simulink model "Test7_withSimscapeBus"  (R2019b)
settings: Solver=VariableStepAuto  StartTime=0.0  StopTime=5  RelTol=1e-3
undefined symbols (not defined in the file): High, Low
libraries: fl_lib x49, nesl_utility x15, ee_lib x4, simulink x1
settings Model: Creator=lenovo  LastModifiedBy=czm6597
settings DebuggingCC: UnconnectedInputMsg=none  UnconnectedOutputMsg=none  UnconnectedLineMsg=none  SFMachineParentedDataDiag=error
settings ModelReferenceCC: EnableRefExpFcnMdlSchedulingChecks=off
settings RTWCC: Description=Generic Real-Time Target

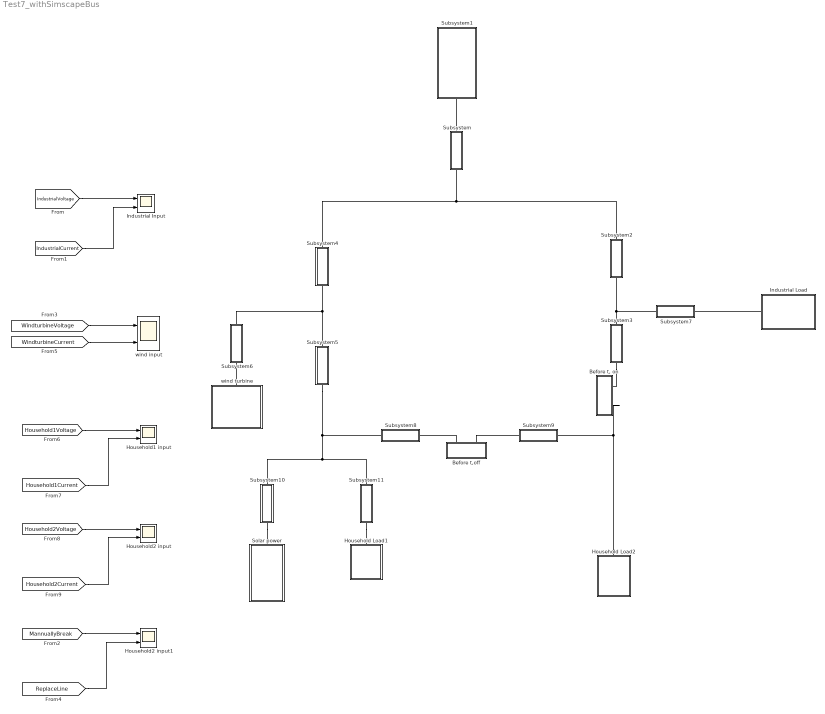
== system Test7_withSimscapeBus ==
  "Before t, on" : Subsystem  mask{t=3}
      mask prompts: t "Specific jumping time"
  Before t,off : Subsystem  mask{t=3}
      mask prompts: t "Specific jumping time"
  Household Load1 : Subsystem
  Household Load2 : Subsystem
  Household1 input : Scope  NumInputPorts=2
  Household2 input : Scope  NumInputPorts=2
  Household2 input1 : Scope  NumInputPorts=2
  Industrial Input : Scope  NumInputPorts=2
  Industrial Load : Subsystem
  Solar power : Subsystem
  Subsystem : Subsystem  mask{rho=1.68e-8, l=2.0, A=1.5e-6}
      mask prompts: rho "Specific resistivity in Ohm*m"; l "Length in m"; A "Cross sectional area in m^2"
  Subsystem1 : Subsystem
  Subsystem10 : Subsystem  mask{rho=1.68e-8, l=2.0, A=1.5e-6}
      mask prompts: rho "Specific resistivity in Ohm*m"; l "Length in m"; A "Cross sectional area in m^2"
  Subsystem11 : Subsystem  mask{rho=1.68e-8, l=2.0, A=1.5e-6}
      mask prompts: rho "Specific resistivity in Ohm*m"; l "Length in m"; A "Cross sectional area in m^2"
  Subsystem2 : Subsystem  mask{rho=1.68e-8, l=2.0, A=1.5e-6}
      mask prompts: rho "Specific resistivity in Ohm*m"; l "Length in m"; A "Cross sectional area in m^2"
  Subsystem3 : Subsystem  mask{rho=1.68e-8, l=2.0, A=1.5e-6}
      mask prompts: rho "Specific resistivity in Ohm*m"; l "Length in m"; A "Cross sectional area in m^2"
  Subsystem4 : Subsystem  mask{rho=1.68e-8, l=2.0, A=1.5e-6}
      mask prompts: rho "Specific resistivity in Ohm*m"; l "Length in m"; A "Cross sectional area in m^2"
  Subsystem5 : Subsystem  mask{rho=1.68e-8, l=2.0, A=1.5e-6}
      mask prompts: rho "Specific resistivity in Ohm*m"; l "Length in m"; A "Cross sectional area in m^2"
  Subsystem6 : Subsystem  mask{rho=1.68e-8, l=2.0, A=1.5e-6}
      mask prompts: rho "Specific resistivity in Ohm*m"; l "Length in m"; A "Cross sectional area in m^2"
  Subsystem7 : Subsystem  mask{rho=1.68e-8, l=2.0, A=1.5e-6}
      mask prompts: rho "Specific resistivity in Ohm*m"; l "Length in m"; A "Cross sectional area in m^2"
  Subsystem8 : Subsystem  mask{rho=1.68e-8, l=2.0, A=1.5e-6}
      mask prompts: rho "Specific resistivity in Ohm*m"; l "Length in m"; A "Cross sectional area in m^2"
  Subsystem9 : Subsystem  mask{rho=1.68e-8, l=2.0, A=1.5e-6}
      mask prompts: rho "Specific resistivity in Ohm*m"; l "Length in m"; A "Cross sectional area in m^2"
  wind input : Scope  NumInputPorts=2
  wind turbine : Subsystem
  wires:
  [Household2Current] -> Household2 input/2
  [Household2Voltage] -> Household2 input/1
  [Household1Current] -> Household1 input/2
  [Household1Voltage] -> Household1 input/1
  [WindturbineCurrent] -> wind input/2
  [IndustrialCurrent] -> Industrial Input/2
  [IndustrialVoltage] -> Industrial Input/1
  [WindturbineVoltage] -> wind input/1
  [MannuallyBreak] -> Household2 input1/1
  [ReplaceLine] -> Household2 input1/2
  connections:
  Subsystem/RConn1 -- Subsystem4/LConn1 -- Subsystem2/LConn1
  Subsystem/LConn1 -- Subsystem1/RConn1
  Subsystem3/LConn1 -- Subsystem7/LConn1 -- Subsystem2/RConn1
  Subsystem5/LConn1 -- Subsystem6/RConn1 -- Subsystem4/RConn1
  wind turbine/LConn1 -- Subsystem6/LConn1
  Industrial Load/RConn1 -- Subsystem7/RConn1
  Subsystem5/RConn1 -- Subsystem11/LConn1 -- Subsystem10/LConn1 -- Subsystem8/RConn1
  Subsystem11/RConn1 -- Household Load1/LConn1
  Subsystem10/RConn1 -- Solar power/LConn1
  Subsystem3/RConn1 -- "Before t, on"/LConn1
  "Before t, on"/LConn2 -- Household Load2/LConn1 -- Subsystem9/LConn1
  Before t,off/LConn1 -- Subsystem8/LConn1
  Before t,off/LConn2 -- Subsystem9/RConn1

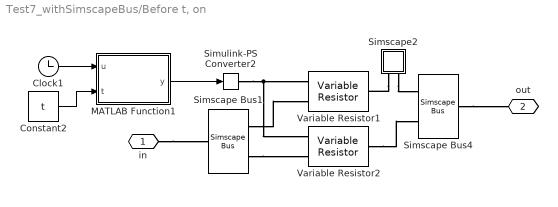
== system Test7_withSimscapeBus/Before t, on ==
  Clock1 : Clock
  Constant2 : Constant  Value=t
  MATLAB Function1 : MATLAB Function  TreatAsAtomicUnit=on
  Simscape Bus1 : SimscapeBus  HierarchyStrings=High;Low
  Simscape Bus4 : SimscapeBus  HierarchyStrings=High;Low
  Simscape2 : Subsystem
      mask Display:
      | disp('A')
      | port_label('LConn',1,'+')
      | port_label('LConn',2,'-')
  Simulink-PS Converter2 : nesl_utility/Simulink-PS Converter  PhysicalDomain=network_engine_domain  SubClassName=ps_input  LeftPortType=input  RightPortType=output  PseudoPeriodic=off  Frequencies=[]  NoiseDistribution=none  NoiseParameters=[]  Unit=1  AffineConversion=off  FilteringAndDerivatives=provide  SimscapeFilterOrder=1  InputFilterTimeConstant=0.001  UdotUserProvided=0
  Variable Resistor1 : fl_lib/Electrical/Electrical Elements/Variable Resistor  Rmin=0 Ohm  i_specify=off  i_priority=None  i=0 A  i_nominal_specify=off  i_nominal_unit=A  i_nominal_value=1  v_specify=off  v_priority=None  v=0 V  v_nominal_specify=off  v_nominal_unit=V  v_nominal_value=1
  Variable Resistor2 : fl_lib/Electrical/Electrical Elements/Variable Resistor  Rmin=0 Ohm  i_specify=off  i_priority=None  i=0 A  i_nominal_specify=off  i_nominal_unit=A  i_nominal_value=1  v_specify=off  v_priority=None  v=0 V  v_nominal_specify=off  v_nominal_unit=V  v_nominal_value=1
  in : PMIOPort  Side=Left
  out : PMIOPort  Port=2  Side=Left
  wires:
  Clock1/1 -> MATLAB Function1/1(u)
  Constant2/1 -> MATLAB Function1/2(t)
  MATLAB Function1/1(y) -> Simulink-PS Converter2/1
  connections:
  Simscape2/LConn1 -- Variable Resistor1/RConn1
  Simulink-PS Converter2/RConn1 -- Variable Resistor1/LConn1 -- Variable Resistor2/LConn1
  in/RConn1 -- Simscape Bus1/RConn1
  Simscape Bus1/LConn2 -- Variable Resistor2/LConn2
  Simscape Bus1/LConn1 -- Variable Resistor1/LConn2
  Variable Resistor2/RConn1 -- Simscape Bus4/LConn2
  Simscape Bus4/RConn1 -- out/RConn1
  Simscape2/LConn2 -- Simscape Bus4/LConn1

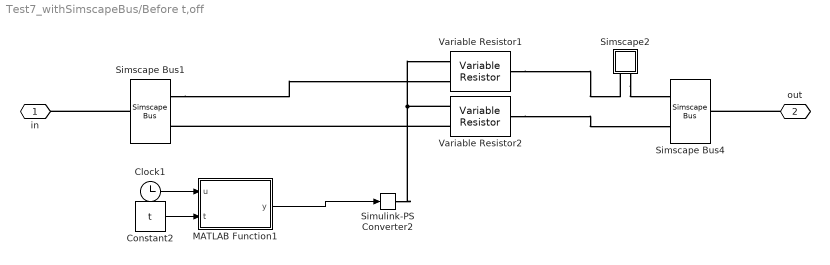
== system Test7_withSimscapeBus/Before t,off ==
  Clock1 : Clock
  Constant2 : Constant  Value=t
  MATLAB Function1 : MATLAB Function  TreatAsAtomicUnit=on
  Simscape Bus1 : SimscapeBus  HierarchyStrings=High;Low
  Simscape Bus4 : SimscapeBus  HierarchyStrings=High;Low
  Simscape2 : Subsystem
      mask Display:
      | disp('A')
      | port_label('LConn',1,'+')
      | port_label('LConn',2,'-')
  Simulink-PS Converter2 : nesl_utility/Simulink-PS Converter  PhysicalDomain=network_engine_domain  SubClassName=ps_input  LeftPortType=input  RightPortType=output  PseudoPeriodic=off  Frequencies=[]  NoiseDistribution=none  NoiseParameters=[]  Unit=1  AffineConversion=off  FilteringAndDerivatives=provide  SimscapeFilterOrder=1  InputFilterTimeConstant=0.001  UdotUserProvided=0
  Variable Resistor1 : fl_lib/Electrical/Electrical Elements/Variable Resistor  Rmin=0 Ohm  i_specify=off  i_priority=None  i=0 A  i_nominal_specify=off  i_nominal_unit=A  i_nominal_value=1  v_specify=off  v_priority=None  v=0 V  v_nominal_specify=off  v_nominal_unit=V  v_nominal_value=1
  Variable Resistor2 : fl_lib/Electrical/Electrical Elements/Variable Resistor  Rmin=0 Ohm  i_specify=off  i_priority=None  i=0 A  i_nominal_specify=off  i_nominal_unit=A  i_nominal_value=1  v_specify=off  v_priority=None  v=0 V  v_nominal_specify=off  v_nominal_unit=V  v_nominal_value=1
  in : PMIOPort  Side=Left
  out : PMIOPort  Port=2  Side=Left
  wires:
  MATLAB Function1/1(y) -> Simulink-PS Converter2/1
  Constant2/1 -> MATLAB Function1/2(t)
  Clock1/1 -> MATLAB Function1/1(u)
  connections:
  out/RConn1 -- Simscape Bus4/RConn1
  Simscape Bus1/RConn1 -- in/RConn1
  Variable Resistor2/LConn2 -- Simscape Bus1/LConn2
  Simscape Bus1/LConn1 -- Variable Resistor1/LConn2
  Variable Resistor1/RConn1 -- Simscape2/LConn1
  Variable Resistor2/RConn1 -- Simscape Bus4/LConn2
  Simulink-PS Converter2/RConn1 -- Variable Resistor1/LConn1 -- Variable Resistor2/LConn1
  Simscape2/LConn2 -- Simscape Bus4/LConn1

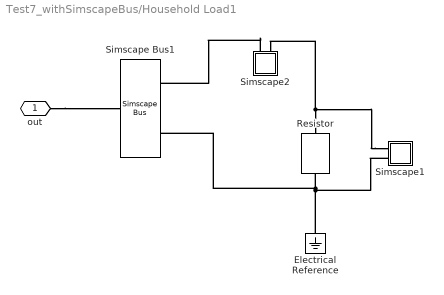
== system Test7_withSimscapeBus/Household Load1 ==
  Electrical Reference : fl_lib/Electrical/Electrical Elements/Electrical Reference
  Resistor : fl_lib/Electrical/Electrical Elements/Resistor  R=1 Ohm  i_specify=off  i_priority=None  i=0 A  i_nominal_specify=off  i_nominal_unit=A  i_nominal_value=1  v_specify=off  v_priority=None  v=0 V  v_nominal_specify=off  v_nominal_unit=V  v_nominal_value=1
  Simscape Bus1 : SimscapeBus  HierarchyStrings=High;Low
  Simscape1 : Subsystem
      mask Display:
      | disp('V')
      | port_label('LConn',1,'+')
      | port_label('LConn',2,'-')
  Simscape2 : Subsystem
      mask Display:
      | disp('A')
      | port_label('LConn',1,'+')
      | port_label('LConn',2,'-')
  out : PMIOPort  Side=Left
  connections:
  Simscape2/LConn1 -- Simscape Bus1/LConn1
  Simscape1/LConn1 -- Simscape2/LConn2 -- Resistor/LConn1
  Simscape1/LConn2 -- Simscape Bus1/LConn2 -- Resistor/RConn1 -- Electrical Reference/LConn1
  out/RConn1 -- Simscape Bus1/RConn1

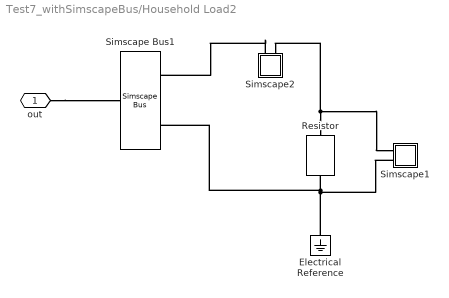
== system Test7_withSimscapeBus/Household Load2 ==
  Electrical Reference : fl_lib/Electrical/Electrical Elements/Electrical Reference
  Resistor : fl_lib/Electrical/Electrical Elements/Resistor  R=1 Ohm  i_specify=off  i_priority=None  i=0 A  i_nominal_specify=off  i_nominal_unit=A  i_nominal_value=1  v_specify=off  v_priority=None  v=0 V  v_nominal_specify=off  v_nominal_unit=V  v_nominal_value=1
  Simscape Bus1 : SimscapeBus  HierarchyStrings=High;Low
  Simscape1 : Subsystem
      mask Display:
      | disp('V')
      | port_label('LConn',1,'+')
      | port_label('LConn',2,'-')
  Simscape2 : Subsystem
      mask Display:
      | disp('A')
      | port_label('LConn',1,'+')
      | port_label('LConn',2,'-')
  out : PMIOPort  Side=Left
  connections:
  Electrical Reference/LConn1 -- Simscape Bus1/LConn2 -- Resistor/RConn1 -- Simscape1/LConn2
  Resistor/LConn1 -- Simscape2/LConn2 -- Simscape1/LConn1
  Simscape2/LConn1 -- Simscape Bus1/LConn1
  out/RConn1 -- Simscape Bus1/RConn1

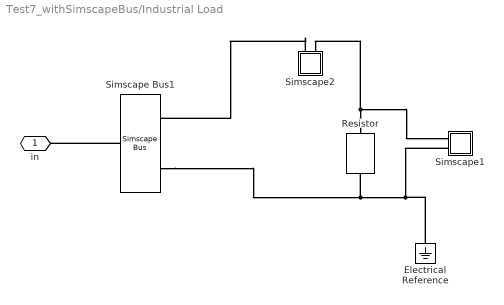
== system Test7_withSimscapeBus/Industrial Load ==
  Electrical Reference : fl_lib/Electrical/Electrical Elements/Electrical Reference
  Resistor : fl_lib/Electrical/Electrical Elements/Resistor  R=1 Ohm  i_specify=off  i_priority=None  i=0 A  i_nominal_specify=off  i_nominal_unit=A  i_nominal_value=1  v_specify=off  v_priority=None  v=0 V  v_nominal_specify=off  v_nominal_unit=V  v_nominal_value=1
  Simscape Bus1 : SimscapeBus  HierarchyStrings=High;Low
  Simscape1 : Subsystem
      mask Display:
      | disp('V')
      | port_label('LConn',1,'+')
      | port_label('LConn',2,'-')
  Simscape2 : Subsystem
      mask Display:
      | disp('A')
      | port_label('LConn',1,'+')
      | port_label('LConn',2,'-')
  in : PMIOPort  Side=Right
  connections:
  Simscape2/LConn1 -- Simscape Bus1/LConn1
  Simscape Bus1/RConn1 -- in/RConn1
  Resistor/LConn1 -- Simscape2/LConn2 -- Simscape1/LConn1
  Electrical Reference/LConn1 -- Simscape Bus1/LConn2 -- Resistor/RConn1 -- Simscape1/LConn2

== system Test7_withSimscapeBus/Solar power ==
  Current Source1 : ee_lib/Sources/Current Source  dc_current=0.6 A  ac_current=0 A  ac_shift=0 rad  ac_frequency=60 Hz  noise_mode=0  PSD=0 A^2/Hz  repeatability=1  auto_seed=2280044724  user_seed=0  sample_time=1e-3 s  i_specify=off  i_priority=None  i=0 A  i_nominal_specify=off  i_nominal_unit=A  i_nominal_value=1  v_specify=off  v_priority=None  v=0 V  v_nominal_specify=off  v_nominal_unit=V  v_nominal_value=1
      settings: SourceProductName=Simscape Electrical  SourceProductBaseCode=PS
  Resistor : ee_lib/Passive/Resistor  R=0.3 Ohm  R_tol=5  enable_R_tol=0  tol_distribution=1  nSigma=4  enable_operating_limits=0  operating_limit_action=2  max_working_voltage=100 V  power_rating=1 W  enable_faults=0  fault_action=1  R_faulted=inf Ohm  enable_temporal_fault=0  t_fault=1 s  enable_behavioral_fault=0  max_permissible_current=1 A  t_fail_on_current=1 s  noise_mode=0  sample_time=1e-3 s  repeatability=1  auto_seed=2715962282  user_seed=0  Tdevice=25 degC  alpha=3.93e-3 1/K  Tmeas=25 degC  thermal_mass=100 J/K  power_derating_T1=70 degC  power_derating_T2=155 degC  operating_temperature_range_vec=[-50, 150] degC  temperature_specify=off  temperature_priority=High  temperature=298.15 K  temperature_nominal_specify=off  temperature_nominal_unit=K  temperature_nominal_value=1
      settings: SourceProductName=Simscape Electrical
  Simscape Bus1 : SimscapeBus  HierarchyStrings=High;Low
  out : PMIOPort  Side=Left
  connections:
  Simscape Bus1/LConn1 -- Current Source1/LConn1 -- Resistor/LConn1
  Resistor/RConn1 -- Current Source1/RConn1 -- Simscape Bus1/LConn2
  out/RConn1 -- Simscape Bus1/RConn1

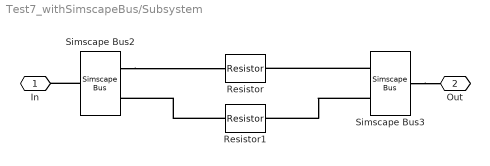
== system Test7_withSimscapeBus/Subsystem ==
  Resistor : fl_lib/Electrical/Electrical Elements/Resistor  R=rho*l/A Ohm  i_specify=off  i_priority=None  i=0 A  i_nominal_specify=off  i_nominal_unit=A  i_nominal_value=1  v_specify=off  v_priority=None  v=0 V  v_nominal_specify=off  v_nominal_unit=V  v_nominal_value=1
  Resistor1 : fl_lib/Electrical/Electrical Elements/Resistor  R=rho*l/A Ohm  i_specify=off  i_priority=None  i=0 A  i_nominal_specify=off  i_nominal_unit=A  i_nominal_value=1  v_specify=off  v_priority=None  v=0 V  v_nominal_specify=off  v_nominal_unit=V  v_nominal_value=1
  Simscape Bus2 : SimscapeBus  HierarchyStrings=High;Low
  Simscape Bus3 : SimscapeBus  HierarchyStrings=High;Low
  In : PMIOPort  Side=Left
  Out : PMIOPort  Port=2  Side=Right
  connections:
  Simscape Bus2/LConn1 -- Resistor/LConn1
  Simscape Bus3/LConn2 -- Resistor1/RConn1
  Simscape Bus2/RConn1 -- In/RConn1
  Simscape Bus3/LConn1 -- Resistor/RConn1
  Resistor1/LConn1 -- Simscape Bus2/LConn2
  Simscape Bus3/RConn1 -- Out/RConn1

== system Test7_withSimscapeBus/Subsystem1 ==
  note: DC voltage source
  note: DLP: DC line parameter
  DC Voltage Source1 : ee_lib/Additional Components/SPICE Sources/DC Voltage Source  DC=5 V
      settings: SourceProductName=Simscape Electrical
  Electrical Reference1 : fl_lib/Electrical/Electrical Elements/Electrical Reference
  Simscape Bus : SimscapeBus  HierarchyStrings=High;Low
  Solver Configuration1 : nesl_utility/Solver Configuration  PhysicalDomain=network_engine_domain  SubClassName=solver  LeftPortType=input  RightPortType=generic  Tones=[]  Harmonics=[]  SimulateNoise=off  Profile=off  UseLocalSampling=off  EnableSwitchedLinearOptims=on  FrequencyDomain=off  UseCCode=off  RelTol=0.001  AbsTol=1e-06  MinStep=1e-09  ToWorkspace=off  RevertToSquareIcSolve=off  NumHomotopyIterations=100  PhasorMode=off  PhasorModeNumHarmonics=1  DoDC=off  ResidualTolerance=1e-9  UseLocalSolver=on  LocalSolverChoice=NE_BACKWARD_EULER_ADVANCER  LocalSolverSampleTime=5e-6  DoFixedCost=on  MaxNonlinIter=3  MaxModeIter=2  LinearAlgebra=auto  EquationFormulation=NE_TIME_EF  DelaysMemoryBudget=1024  AutomaticFiltering=on  FilteringTimeConstant=0.001  PartitionStorageMethod=AS_NEEDED  PartitionMemoryBudget=1024  PartitionMethod=FAST
  out : PMIOPort  Side=Right
  connections:
  DC Voltage Source1/LConn1 -- Simscape Bus/LConn1
  DC Voltage Source1/RConn1 -- Simscape Bus/LConn2 -- Electrical Reference1/LConn1 -- Solver Configuration1/RConn1
  out/RConn1 -- Simscape Bus/RConn1

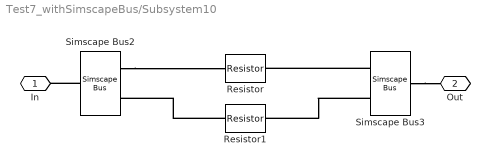
== system Test7_withSimscapeBus/Subsystem10 ==
  Resistor : fl_lib/Electrical/Electrical Elements/Resistor  R=rho*l/A Ohm  i_specify=off  i_priority=None  i=0 A  i_nominal_specify=off  i_nominal_unit=A  i_nominal_value=1  v_specify=off  v_priority=None  v=0 V  v_nominal_specify=off  v_nominal_unit=V  v_nominal_value=1
  Resistor1 : fl_lib/Electrical/Electrical Elements/Resistor  R=rho*l/A Ohm  i_specify=off  i_priority=None  i=0 A  i_nominal_specify=off  i_nominal_unit=A  i_nominal_value=1  v_specify=off  v_priority=None  v=0 V  v_nominal_specify=off  v_nominal_unit=V  v_nominal_value=1
  Simscape Bus2 : SimscapeBus  HierarchyStrings=High;Low
  Simscape Bus3 : SimscapeBus  HierarchyStrings=High;Low
  In : PMIOPort  Side=Left
  Out : PMIOPort  Port=2  Side=Right
  connections:
  Simscape Bus3/RConn1 -- Out/RConn1
  Resistor1/LConn1 -- Simscape Bus2/LConn2
  Simscape Bus3/LConn1 -- Resistor/RConn1
  Simscape Bus2/RConn1 -- In/RConn1
  Simscape Bus3/LConn2 -- Resistor1/RConn1
  Simscape Bus2/LConn1 -- Resistor/LConn1

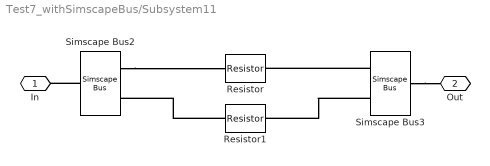
== system Test7_withSimscapeBus/Subsystem11 ==
  Resistor : fl_lib/Electrical/Electrical Elements/Resistor  R=rho*l/A Ohm  i_specify=off  i_priority=None  i=0 A  i_nominal_specify=off  i_nominal_unit=A  i_nominal_value=1  v_specify=off  v_priority=None  v=0 V  v_nominal_specify=off  v_nominal_unit=V  v_nominal_value=1
  Resistor1 : fl_lib/Electrical/Electrical Elements/Resistor  R=rho*l/A Ohm  i_specify=off  i_priority=None  i=0 A  i_nominal_specify=off  i_nominal_unit=A  i_nominal_value=1  v_specify=off  v_priority=None  v=0 V  v_nominal_specify=off  v_nominal_unit=V  v_nominal_value=1
  Simscape Bus2 : SimscapeBus  HierarchyStrings=High;Low
  Simscape Bus3 : SimscapeBus  HierarchyStrings=High;Low
  In : PMIOPort  Side=Left
  Out : PMIOPort  Port=2  Side=Right
  connections:
  Simscape Bus2/LConn1 -- Resistor/LConn1
  Simscape Bus3/LConn2 -- Resistor1/RConn1
  Simscape Bus2/RConn1 -- In/RConn1
  Simscape Bus3/LConn1 -- Resistor/RConn1
  Resistor1/LConn1 -- Simscape Bus2/LConn2
  Simscape Bus3/RConn1 -- Out/RConn1

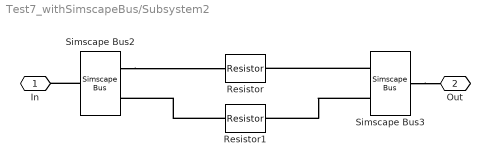
== system Test7_withSimscapeBus/Subsystem2 ==
  Resistor : fl_lib/Electrical/Electrical Elements/Resistor  R=rho*l/A Ohm  i_specify=off  i_priority=None  i=0 A  i_nominal_specify=off  i_nominal_unit=A  i_nominal_value=1  v_specify=off  v_priority=None  v=0 V  v_nominal_specify=off  v_nominal_unit=V  v_nominal_value=1
  Resistor1 : fl_lib/Electrical/Electrical Elements/Resistor  R=rho*l/A Ohm  i_specify=off  i_priority=None  i=0 A  i_nominal_specify=off  i_nominal_unit=A  i_nominal_value=1  v_specify=off  v_priority=None  v=0 V  v_nominal_specify=off  v_nominal_unit=V  v_nominal_value=1
  Simscape Bus2 : SimscapeBus  HierarchyStrings=High;Low
  Simscape Bus3 : SimscapeBus  HierarchyStrings=High;Low
  In : PMIOPort  Side=Left
  Out : PMIOPort  Port=2  Side=Right
  connections:
  Simscape Bus3/RConn1 -- Out/RConn1
  Resistor1/LConn1 -- Simscape Bus2/LConn2
  Simscape Bus3/LConn1 -- Resistor/RConn1
  Simscape Bus2/RConn1 -- In/RConn1
  Simscape Bus3/LConn2 -- Resistor1/RConn1
  Simscape Bus2/LConn1 -- Resistor/LConn1

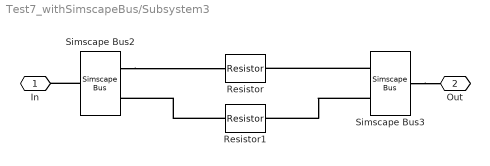
== system Test7_withSimscapeBus/Subsystem3 ==
  Resistor : fl_lib/Electrical/Electrical Elements/Resistor  R=rho*l/A Ohm  i_specify=off  i_priority=None  i=0 A  i_nominal_specify=off  i_nominal_unit=A  i_nominal_value=1  v_specify=off  v_priority=None  v=0 V  v_nominal_specify=off  v_nominal_unit=V  v_nominal_value=1
  Resistor1 : fl_lib/Electrical/Electrical Elements/Resistor  R=rho*l/A Ohm  i_specify=off  i_priority=None  i=0 A  i_nominal_specify=off  i_nominal_unit=A  i_nominal_value=1  v_specify=off  v_priority=None  v=0 V  v_nominal_specify=off  v_nominal_unit=V  v_nominal_value=1
  Simscape Bus2 : SimscapeBus  HierarchyStrings=High;Low
  Simscape Bus3 : SimscapeBus  HierarchyStrings=High;Low
  In : PMIOPort  Side=Left
  Out : PMIOPort  Port=2  Side=Right
  connections:
  Simscape Bus3/RConn1 -- Out/RConn1
  Resistor1/LConn1 -- Simscape Bus2/LConn2
  Simscape Bus3/LConn1 -- Resistor/RConn1
  Simscape Bus2/RConn1 -- In/RConn1
  Simscape Bus3/LConn2 -- Resistor1/RConn1
  Simscape Bus2/LConn1 -- Resistor/LConn1

== system Test7_withSimscapeBus/Subsystem4 ==
  Resistor : fl_lib/Electrical/Electrical Elements/Resistor  R=rho*l/A Ohm  i_specify=off  i_priority=None  i=0 A  i_nominal_specify=off  i_nominal_unit=A  i_nominal_value=1  v_specify=off  v_priority=None  v=0 V  v_nominal_specify=off  v_nominal_unit=V  v_nominal_value=1
  Resistor1 : fl_lib/Electrical/Electrical Elements/Resistor  R=rho*l/A Ohm  i_specify=off  i_priority=None  i=0 A  i_nominal_specify=off  i_nominal_unit=A  i_nominal_value=1  v_specify=off  v_priority=None  v=0 V  v_nominal_specify=off  v_nominal_unit=V  v_nominal_value=1
  Simscape Bus2 : SimscapeBus  HierarchyStrings=High;Low
  Simscape Bus3 : SimscapeBus  HierarchyStrings=High;Low
  In : PMIOPort  Side=Left
  Out : PMIOPort  Port=2  Side=Right
  connections:
  Simscape Bus3/RConn1 -- Out/RConn1
  Resistor1/LConn1 -- Simscape Bus2/LConn2
  Simscape Bus3/LConn1 -- Resistor/RConn1
  Simscape Bus2/RConn1 -- In/RConn1
  Simscape Bus3/LConn2 -- Resistor1/RConn1
  Simscape Bus2/LConn1 -- Resistor/LConn1

== system Test7_withSimscapeBus/Subsystem5 ==
  Resistor : fl_lib/Electrical/Electrical Elements/Resistor  R=rho*l/A Ohm  i_specify=off  i_priority=None  i=0 A  i_nominal_specify=off  i_nominal_unit=A  i_nominal_value=1  v_specify=off  v_priority=None  v=0 V  v_nominal_specify=off  v_nominal_unit=V  v_nominal_value=1
  Resistor1 : fl_lib/Electrical/Electrical Elements/Resistor  R=rho*l/A Ohm  i_specify=off  i_priority=None  i=0 A  i_nominal_specify=off  i_nominal_unit=A  i_nominal_value=1  v_specify=off  v_priority=None  v=0 V  v_nominal_specify=off  v_nominal_unit=V  v_nominal_value=1
  Simscape Bus2 : SimscapeBus  HierarchyStrings=High;Low
  Simscape Bus3 : SimscapeBus  HierarchyStrings=High;Low
  In : PMIOPort  Side=Left
  Out : PMIOPort  Port=2  Side=Right
  connections:
  Simscape Bus2/LConn1 -- Resistor/LConn1
  Simscape Bus3/LConn2 -- Resistor1/RConn1
  Simscape Bus2/RConn1 -- In/RConn1
  Simscape Bus3/LConn1 -- Resistor/RConn1
  Resistor1/LConn1 -- Simscape Bus2/LConn2
  Simscape Bus3/RConn1 -- Out/RConn1

== system Test7_withSimscapeBus/Subsystem6 ==
  Resistor : fl_lib/Electrical/Electrical Elements/Resistor  R=rho*l/A Ohm  i_specify=off  i_priority=None  i=0 A  i_nominal_specify=off  i_nominal_unit=A  i_nominal_value=1  v_specify=off  v_priority=None  v=0 V  v_nominal_specify=off  v_nominal_unit=V  v_nominal_value=1
  Resistor1 : fl_lib/Electrical/Electrical Elements/Resistor  R=rho*l/A Ohm  i_specify=off  i_priority=None  i=0 A  i_nominal_specify=off  i_nominal_unit=A  i_nominal_value=1  v_specify=off  v_priority=None  v=0 V  v_nominal_specify=off  v_nominal_unit=V  v_nominal_value=1
  Simscape Bus2 : SimscapeBus  HierarchyStrings=High;Low
  Simscape Bus3 : SimscapeBus  HierarchyStrings=High;Low
  In : PMIOPort  Side=Left
  Out : PMIOPort  Port=2  Side=Right
  connections:
  Simscape Bus2/LConn1 -- Resistor/LConn1
  Simscape Bus3/LConn2 -- Resistor1/RConn1
  Simscape Bus2/RConn1 -- In/RConn1
  Simscape Bus3/LConn1 -- Resistor/RConn1
  Resistor1/LConn1 -- Simscape Bus2/LConn2
  Simscape Bus3/RConn1 -- Out/RConn1

== system Test7_withSimscapeBus/Subsystem7 ==
  Resistor : fl_lib/Electrical/Electrical Elements/Resistor  R=rho*l/A Ohm  i_specify=off  i_priority=None  i=0 A  i_nominal_specify=off  i_nominal_unit=A  i_nominal_value=1  v_specify=off  v_priority=None  v=0 V  v_nominal_specify=off  v_nominal_unit=V  v_nominal_value=1
  Resistor1 : fl_lib/Electrical/Electrical Elements/Resistor  R=rho*l/A Ohm  i_specify=off  i_priority=None  i=0 A  i_nominal_specify=off  i_nominal_unit=A  i_nominal_value=1  v_specify=off  v_priority=None  v=0 V  v_nominal_specify=off  v_nominal_unit=V  v_nominal_value=1
  Simscape Bus2 : SimscapeBus  HierarchyStrings=High;Low
  Simscape Bus3 : SimscapeBus  HierarchyStrings=High;Low
  In : PMIOPort  Side=Left
  Out : PMIOPort  Port=2  Side=Right
  connections:
  Simscape Bus2/LConn1 -- Resistor/LConn1
  Simscape Bus3/LConn2 -- Resistor1/RConn1
  Simscape Bus2/RConn1 -- In/RConn1
  Simscape Bus3/LConn1 -- Resistor/RConn1
  Resistor1/LConn1 -- Simscape Bus2/LConn2
  Simscape Bus3/RConn1 -- Out/RConn1

== system Test7_withSimscapeBus/Subsystem8 ==
  Resistor : fl_lib/Electrical/Electrical Elements/Resistor  R=rho*l/A Ohm  i_specify=off  i_priority=None  i=0 A  i_nominal_specify=off  i_nominal_unit=A  i_nominal_value=1  v_specify=off  v_priority=None  v=0 V  v_nominal_specify=off  v_nominal_unit=V  v_nominal_value=1
  Resistor1 : fl_lib/Electrical/Electrical Elements/Resistor  R=rho*l/A Ohm  i_specify=off  i_priority=None  i=0 A  i_nominal_specify=off  i_nominal_unit=A  i_nominal_value=1  v_specify=off  v_priority=None  v=0 V  v_nominal_specify=off  v_nominal_unit=V  v_nominal_value=1
  Simscape Bus2 : SimscapeBus  HierarchyStrings=High;Low
  Simscape Bus3 : SimscapeBus  HierarchyStrings=High;Low
  In : PMIOPort  Side=Left
  Out : PMIOPort  Port=2  Side=Right
  connections:
  Simscape Bus3/RConn1 -- Out/RConn1
  Resistor1/LConn1 -- Simscape Bus2/LConn2
  Simscape Bus3/LConn1 -- Resistor/RConn1
  Simscape Bus2/RConn1 -- In/RConn1
  Simscape Bus3/LConn2 -- Resistor1/RConn1
  Simscape Bus2/LConn1 -- Resistor/LConn1

== system Test7_withSimscapeBus/Subsystem9 ==
  Resistor : fl_lib/Electrical/Electrical Elements/Resistor  R=rho*l/A Ohm  i_specify=off  i_priority=None  i=0 A  i_nominal_specify=off  i_nominal_unit=A  i_nominal_value=1  v_specify=off  v_priority=None  v=0 V  v_nominal_specify=off  v_nominal_unit=V  v_nominal_value=1
  Resistor1 : fl_lib/Electrical/Electrical Elements/Resistor  R=rho*l/A Ohm  i_specify=off  i_priority=None  i=0 A  i_nominal_specify=off  i_nominal_unit=A  i_nominal_value=1  v_specify=off  v_priority=None  v=0 V  v_nominal_specify=off  v_nominal_unit=V  v_nominal_value=1
  Simscape Bus2 : SimscapeBus  HierarchyStrings=High;Low
  Simscape Bus3 : SimscapeBus  HierarchyStrings=High;Low
  In : PMIOPort  Side=Left
  Out : PMIOPort  Port=2  Side=Right
  connections:
  Simscape Bus2/LConn1 -- Resistor/LConn1
  Simscape Bus3/LConn2 -- Resistor1/RConn1
  Simscape Bus2/RConn1 -- In/RConn1
  Simscape Bus3/LConn1 -- Resistor/RConn1
  Resistor1/LConn1 -- Simscape Bus2/LConn2
  Simscape Bus3/RConn1 -- Out/RConn1

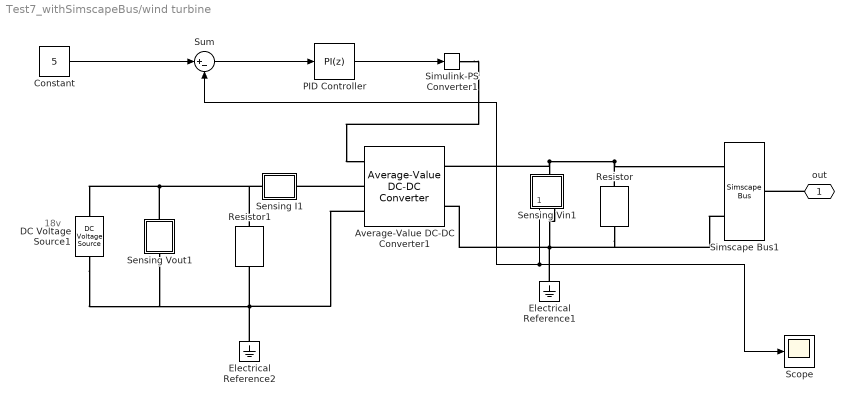
== system Test7_withSimscapeBus/wind turbine ==
  note: 18v
  Average-Value DC-DC Converter1 : ee_lib/Semiconductors & Converters/Converters/Average-Value DC-DC Converter  converter_type=1
      settings: SourceProductName=Simscape Electrical  SourceProductBaseCode=PS  InternalSimscapePortConfiguration="{\"Bottom\":[],\"Left\":[{\"id\":\"DutyCycle\",\"label\":\"DutyCycle\",\"type\":\"input\"},{\"id\":\"p1\",\"label\":\"1+\",\"type\":\"foundation.electrical.electrical\"},{\"id\":\"n1\",\"label\":\"1-\",\"type\":\"foundation.electrical.electrical\"}],\"Right\":[{\"id\":\"p2\",\"label\":\"2+\",\"type\":\"foundation.electrical.electrical\"},{\"id\":\"n2\",\"label\":\"2-\",\"type\":\"foundation.electrical.electrical\"}],\"Top\":[]}"
  Constant : Constant  Value=5
  DC Voltage Source1 : fl_lib/Electrical/Electrical Sources/DC Voltage Source  v0=18 V
  Electrical Reference1 : fl_lib/Electrical/Electrical Elements/Electrical Reference
  Electrical Reference2 : fl_lib/Electrical/Electrical Elements/Electrical Reference
  PID Controller : simulink/Continuous/PID Controller  Controller=PI  Form=Parallel  TimeDomain=Discrete-time  SampleTime=1e-6  IntegratorMethod=Forward Euler  FilterMethod=Forward Euler  ControllerParametersSource=internal  P=1.75265929022857e-07  I=0.350531858045715  D=0  UseFilter=on  N=100  TunerSelectOption=Transfer Function Based (PID Tuner App)  InitialConditionSource=internal  InitialConditionForIntegrator=0.53  InitialConditionForFilter=0  DifferentiatorICPrevScaledInput=0  ExternalReset=none  TrackingMode=off  Kt=1  LimitOutput=on  UpperSaturationLimit=0.99  LowerSaturationLimit=0.16  LinearizeAsGain=off  AntiWindupMode=none  Kb=1  POutMin=[]  POutMax=[]  IOutMin=[]  IOutMax=[]  DOutMin=[]  DOutMax=[]  NOutMin=[]  NOutMax=[]  SumOutMin=[]  SumOutMax=[]  SaturationOutMin=[]  SaturationOutMax=[]  PParamMin=[]  PParamMax=[]  IParamMin=[]  IParamMax=[]  DParamMin=[]  DParamMax=[]  NParamMin=[]  NParamMax=[]  KbParamMin=[]  KbParamMax=[]  KtParamMin=[]  KtParamMax=[]  KbOutMin=[]  KbOutMax=[]  KtOutMin=[]  KtOutMax=[]  IntegratorOutMin=[]  IntegratorOutMax=[]  FilterOutMin=[]  FilterOutMax=[]  SumI1OutMin=[]  SumI1OutMax=[]  SumI2OutMin=[]  SumI2OutMax=[]  SumI3OutMin=[]  SumI3OutMax=[]  SumI4OutMin=[]  SumI4OutMax=[]  SumDOutMin=[]  SumDOutMax=[]  DifferentiatorOutMin=[]  DifferentiatorOutMax=[]  FilterDiffOutCoefMin=[]  FilterDiffOutCoefMax=[]  ReciprocalOutMin=[]  ReciprocalOutMax=[]  SumDenOutMin=[]  SumDenOutMax=[]  SumNumOutMin=[]  SumNumOutMax=[]  DivideOutMin=[]  DivideOutMax=[]  IntegratorContinuousStateAttributes=''  IntegratorStateMustResolveToSignalObject=off  IntegratorRTWStateStorageClass=Auto  FilterContinuousStateAttributes=''  FilterStateMustResolveToSignalObject=off  FilterRTWStateStorageClass=Auto  ParallelPVariant=InternalParameters  IdealPVariant=Disabled  IVariant=InternalParameters  DVariant=Disabled  IntegratorVariant=Discrete  SatVariant=Enabled  AWVariant=Passthrough  PCopyVariant=Disabled  TRVariant=Disabled  FdbkBlocksVariant=Forward  IdealPFdbkVariant=Disabled  SatFdbkVariant=Disabled  DerivativeFilterVariant=Disabled  NVariant=Disabled  NCopyVariant=Disabled_SignalSpec  FilterICVariant=Disabled  IntegratorICVariant=InternalICs  ExternalResetVariant=Disabled  TRSumVariant=Passthrough  SumFdbkVariant=Disabled  SumVariant=Sum_PI
  Resistor : fl_lib/Electrical/Electrical Elements/Resistor  R=1 Ohm  i_specify=off  i_priority=None  i=0 A  i_nominal_specify=off  i_nominal_unit=A  i_nominal_value=1  v_specify=off  v_priority=None  v=0 V  v_nominal_specify=off  v_nominal_unit=V  v_nominal_value=1
  Resistor1 : fl_lib/Electrical/Electrical Elements/Resistor  R=50 Ohm  i_specify=off  i_priority=None  i=0 A  i_nominal_specify=off  i_nominal_unit=A  i_nominal_value=1  v_specify=off  v_priority=None  v=0 V  v_nominal_specify=off  v_nominal_unit=V  v_nominal_value=1
  Scope : Scope
  Sensing Vin1 : Subsystem
      mask Display:
      | disp('V')
      | port_label('Lconn',1,'+')
      | port_label('Rconn',1,'-')
  Sensing Vout1 : Subsystem
      mask Display:
      | disp('V')
      | port_label('Lconn',1,'+')
      | port_label('Rconn',1,'-')
  Sensing I1 : Subsystem
      mask Display:
      | disp('I')
      | port_label('Lconn',1,'+')
      | port_label('Rconn',1,'-')
  Simscape Bus1 : SimscapeBus  HierarchyStrings=High;Low
  Simulink-PS Converter1 : nesl_utility/Simulink-PS Converter  PhysicalDomain=network_engine_domain  SubClassName=ps_input  LeftPortType=input  RightPortType=output  PseudoPeriodic=off  Frequencies=[]  NoiseDistribution=none  NoiseParameters=[]  Unit=1  AffineConversion=off  FilteringAndDerivatives=provide  SimscapeFilterOrder=1  InputFilterTimeConstant=0.001  UdotUserProvided=0
  Sum : Sum  Inputs=|+-
  out : PMIOPort  Side=Left
  wires:
  Sensing Vin1/1(Vout) -> Scope/1, Sum/2
  Constant/1 -> Sum/1
  Sum/1 -> PID Controller/1
  PID Controller/1 -> Simulink-PS Converter1/1
  connections:
  Sensing Vin1/RConn1 -- Average-Value DC-DC Converter1/RConn2 -- Resistor/RConn1 -- Simscape Bus1/LConn2 -- Electrical Reference1/LConn1
  Sensing Vin1/LConn1 -- Average-Value DC-DC Converter1/RConn1 -- Resistor/LConn1 -- Simscape Bus1/LConn1
  Sensing Vout1/RConn1 -- DC Voltage Source1/RConn1 -- Average-Value DC-DC Converter1/LConn3 -- Electrical Reference2/LConn1 -- Resistor1/RConn1
  Sensing Vout1/LConn1 -- DC Voltage Source1/LConn1 -- Resistor1/LConn1 -- Sensing I1/LConn1
  Average-Value DC-DC Converter1/LConn2 -- Sensing I1/RConn1
  out/RConn1 -- Simscape Bus1/RConn1
  Simulink-PS Converter1/RConn1 -- Average-Value DC-DC Converter1/LConn1

== system Test7_withSimscapeBus/Before t, on/Simscape2 ==
  Current Sensor : fl_lib/Electrical/Electrical Sensors/Current Sensor
  PS-S : nesl_utility/PS-Simulink Converter  PhysicalDomain=network_engine_domain  SubClassName=ps_output  LeftPortType=input  RightPortType=output  PseudoPeriodic=off  Frequencies=[]  Unit=A  AffineConversion=off
  + : PMIOPort  Side=Left
  - : PMIOPort  Port=2  Side=Left
  tag scope: MannuallyBreak=global
  wires:
  PS-S/1 -> [MannuallyBreak]  "current"
  connections:
  PS-S/LConn1 -- Current Sensor/RConn1
  Current Sensor/LConn1 -- +/RConn1
  -/RConn1 -- Current Sensor/RConn2

== system Test7_withSimscapeBus/Before t,off/Simscape2 ==
  Current Sensor : fl_lib/Electrical/Electrical Sensors/Current Sensor
  PS-S : nesl_utility/PS-Simulink Converter  PhysicalDomain=network_engine_domain  SubClassName=ps_output  LeftPortType=input  RightPortType=output  PseudoPeriodic=off  Frequencies=[]  Unit=A  AffineConversion=off
  + : PMIOPort  Side=Left
  - : PMIOPort  Port=2  Side=Left
  tag scope: ReplaceLine=global
  wires:
  PS-S/1 -> [ReplaceLine]  "current"
  connections:
  PS-S/LConn1 -- Current Sensor/RConn1
  Current Sensor/LConn1 -- +/RConn1
  -/RConn1 -- Current Sensor/RConn2

== system Test7_withSimscapeBus/Household Load1/Simscape1 ==
  PS-S : nesl_utility/PS-Simulink Converter  PhysicalDomain=network_engine_domain  SubClassName=ps_output  LeftPortType=input  RightPortType=output  PseudoPeriodic=off  Frequencies=[]  Unit=V  AffineConversion=off
  Voltage Sensor : fl_lib/Electrical/Electrical Sensors/Voltage Sensor
  + : PMIOPort  Side=Left
  - : PMIOPort  Port=2  Side=Left
  tag scope: Household1Voltage=global
  wires:
  PS-S/1 -> [Household1Voltage]  "voltage"
  connections:
  PS-S/LConn1 -- Voltage Sensor/RConn1
  +/RConn1 -- Voltage Sensor/LConn1
  Voltage Sensor/RConn2 -- -/RConn1

== system Test7_withSimscapeBus/Household Load1/Simscape2 ==
  Current Sensor : fl_lib/Electrical/Electrical Sensors/Current Sensor
  PS-S : nesl_utility/PS-Simulink Converter  PhysicalDomain=network_engine_domain  SubClassName=ps_output  LeftPortType=input  RightPortType=output  PseudoPeriodic=off  Frequencies=[]  Unit=A  AffineConversion=off
  + : PMIOPort  Side=Left
  - : PMIOPort  Port=2  Side=Left
  tag scope: Household1Current=global
  wires:
  PS-S/1 -> [Household1Current]  "current"
  connections:
  -/RConn1 -- Current Sensor/RConn2
  Current Sensor/LConn1 -- +/RConn1
  PS-S/LConn1 -- Current Sensor/RConn1

== system Test7_withSimscapeBus/Household Load2/Simscape1 ==
  PS-S : nesl_utility/PS-Simulink Converter  PhysicalDomain=network_engine_domain  SubClassName=ps_output  LeftPortType=input  RightPortType=output  PseudoPeriodic=off  Frequencies=[]  Unit=V  AffineConversion=off
  Voltage Sensor : fl_lib/Electrical/Electrical Sensors/Voltage Sensor
  + : PMIOPort  Side=Left
  - : PMIOPort  Port=2  Side=Left
  tag scope: Household2Voltage=global
  wires:
  PS-S/1 -> [Household2Voltage]  "voltage"
  connections:
  Voltage Sensor/RConn2 -- -/RConn1
  +/RConn1 -- Voltage Sensor/LConn1
  PS-S/LConn1 -- Voltage Sensor/RConn1

== system Test7_withSimscapeBus/Household Load2/Simscape2 ==
  Current Sensor : fl_lib/Electrical/Electrical Sensors/Current Sensor
  PS-S : nesl_utility/PS-Simulink Converter  PhysicalDomain=network_engine_domain  SubClassName=ps_output  LeftPortType=input  RightPortType=output  PseudoPeriodic=off  Frequencies=[]  Unit=A  AffineConversion=off
  + : PMIOPort  Side=Left
  - : PMIOPort  Port=2  Side=Left
  tag scope: Household2Current=global
  wires:
  PS-S/1 -> [Household2Current]  "current"
  connections:
  PS-S/LConn1 -- Current Sensor/RConn1
  Current Sensor/LConn1 -- +/RConn1
  -/RConn1 -- Current Sensor/RConn2

== system Test7_withSimscapeBus/Industrial Load/Simscape1 ==
  PS-S : nesl_utility/PS-Simulink Converter  PhysicalDomain=network_engine_domain  SubClassName=ps_output  LeftPortType=input  RightPortType=output  PseudoPeriodic=off  Frequencies=[]  Unit=V  AffineConversion=off
  Voltage Sensor : fl_lib/Electrical/Electrical Sensors/Voltage Sensor
  + : PMIOPort  Side=Left
  - : PMIOPort  Port=2  Side=Left
  tag scope: IndustrialVoltage=global
  wires:
  PS-S/1 -> [IndustrialVoltage]  "voltage"
  connections:
  Voltage Sensor/RConn2 -- -/RConn1
  +/RConn1 -- Voltage Sensor/LConn1
  PS-S/LConn1 -- Voltage Sensor/RConn1

== system Test7_withSimscapeBus/Industrial Load/Simscape2 ==
  Current Sensor : fl_lib/Electrical/Electrical Sensors/Current Sensor
  PS-S : nesl_utility/PS-Simulink Converter  PhysicalDomain=network_engine_domain  SubClassName=ps_output  LeftPortType=input  RightPortType=output  PseudoPeriodic=off  Frequencies=[]  Unit=A  AffineConversion=off
  + : PMIOPort  Side=Left
  - : PMIOPort  Port=2  Side=Left
  tag scope: IndustrialCurrent=global
  wires:
  PS-S/1 -> [IndustrialCurrent]  "current"
  connections:
  PS-S/LConn1 -- Current Sensor/RConn1
  Current Sensor/LConn1 -- +/RConn1
  -/RConn1 -- Current Sensor/RConn2

== system Test7_withSimscapeBus/wind turbine/Sensing Vin1 ==
  PS-Simulink Converter4 : nesl_utility/PS-Simulink Converter  PhysicalDomain=network_engine_domain  SubClassName=ps_output  LeftPortType=input  RightPortType=output  PseudoPeriodic=off  Frequencies=[]  Unit=V  AffineConversion=off
  Voltage Sensor : fl_lib/Electrical/Electrical Sensors/Voltage Sensor
  + : PMIOPort  Side=Left
  - : PMIOPort  Port=2  Side=Right
  Vout : Outport
  wires:
  PS-Simulink Converter4/1 -> Vout/1  "Voltage"
  connections:
  Voltage Sensor/LConn1 -- +/RConn1
  Voltage Sensor/RConn2 -- -/RConn1
  PS-Simulink Converter4/LConn1 -- Voltage Sensor/RConn1

== system Test7_withSimscapeBus/wind turbine/Sensing Vout1 ==
  PS-Simulink Converter4 : nesl_utility/PS-Simulink Converter  PhysicalDomain=network_engine_domain  SubClassName=ps_output  LeftPortType=input  RightPortType=output  PseudoPeriodic=off  Frequencies=[]  Unit=V  AffineConversion=off
  Voltage Sensor : fl_lib/Electrical/Electrical Sensors/Voltage Sensor
  + : PMIOPort  Side=Left
  - : PMIOPort  Port=2  Side=Right
  tag scope: WindturbineVoltage=global
  wires:
  PS-Simulink Converter4/1 -> [WindturbineVoltage]  "voltage"
  connections:
  Voltage Sensor/LConn1 -- +/RConn1
  Voltage Sensor/RConn2 -- -/RConn1
  PS-Simulink Converter4/LConn1 -- Voltage Sensor/RConn1

== system Test7_withSimscapeBus/wind turbine/Sensing I1 ==
  Current Sensor : fl_lib/Electrical/Electrical Sensors/Current Sensor
  PS-Simulink Converter3 : nesl_utility/PS-Simulink Converter  PhysicalDomain=network_engine_domain  SubClassName=ps_output  LeftPortType=input  RightPortType=output  PseudoPeriodic=off  Frequencies=[]  Unit=A  AffineConversion=off
  + : PMIOPort  Side=Left
  - : PMIOPort  Port=2  Side=Right
  tag scope: WindturbineCurrent=global
  wires:
  PS-Simulink Converter3/1 -> [WindturbineCurrent]  "Current"
  connections:
  Current Sensor/RConn2 -- -/RConn1
  Current Sensor/LConn1 -- +/RConn1
  Current Sensor/RConn1 -- PS-Simulink Converter3/LConn1

== matlab function Test7_withSimscapeBus/Before t,off/MATLAB Function1 ==
  data: u input; y output; t input
function y = fcn(u,t)

y = -tanh(10000*(u-t))*1e6+1e6+1e-6;

== matlab function Test7_withSimscapeBus/Before t, on/MATLAB Function1 ==
  data: u input; y output; t input
function y = fcn(u,t)

y = tanh(10000*(u-t))*1e6+1e6+1e-6;
